simulink model "airspeed_throttle_loop"  (R2016a)
settings: Solver=VariableStepAuto  StartTime=0.0  StopTime=10.0  RelTol=1e-3
values from neighbouring files (symbols this model uses):
  a_V1 = 0.4039    [tune_arispeed_throttle.m]
  a_V2 = 6.4361    [tune_arispeed_throttle.m]
  v_ki = wn_airspeed_throttle^2 / a_V2    (= 0.155373595811)    [tune_arispeed_throttle.m]
  v_kp = (2 * zeta_airspeed_throttle * wn_airspeed_throttle - a_V1) / a_V2    (= 0.123692919625)    [tune_arispeed_throttle.m]
settings Model: Creator=andreanv  LastModifiedBy=andreanv

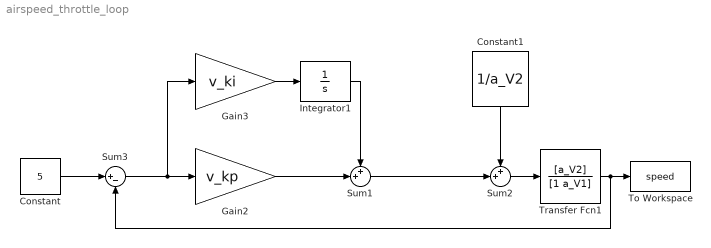
== system airspeed_throttle_loop ==
  Constant : Constant  Value=5
  Constant1 : Constant  Value=1/a_V2
  Gain2 : Gain  Gain=v_kp
  Gain3 : Gain  Gain=v_ki
  Integrator1 : Integrator
  Sum1 : Sum  Inputs=++|
  Sum2 : Sum  Inputs=++|
  Sum3 : Sum  Inputs=|+-
  To Workspace : ToWorkspace  VariableName=speed  SaveFormat=Timeseries  SampleTime=-1
  Transfer Fcn1 : TransferFcn  Numerator=[a_V2]  Denominator=[1 a_V1]
  wires:
  Sum2/1 -> Transfer Fcn1/1
  Transfer Fcn1/1 -> Sum3/2, To Workspace/1
  Gain2/1 -> Sum1/2
  Gain3/1 -> Integrator1/1
  Integrator1/1 -> Sum1/1
  Constant/1 -> Sum3/1
  Sum3/1 -> Gain3/1, Gain2/1
  Sum1/1 -> Sum2/2
  Constant1/1 -> Sum2/1
